simulink library "LiBatteryElements_lib"  (Simulink 7.6)
settings: Solver=ode45  StartTime=0.0  StopTime=10.0  RelTol=1e-3
undefined symbols (not defined in the file or in its folder): gcbh, nesl_callback
settings Model: Creator=rjackey  LastModifiedBy=rjackey

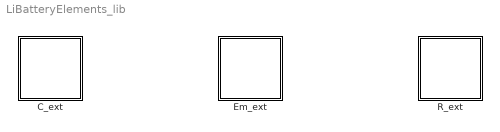
== system LiBatteryElements_lib ==
  C_ext : Subsystem  DialogController=NetworkEngine.DynNeDlgSource  LoadFcn=nesl_callback('LoadFcn',gcbh);  mask(C_ext){ComponentPath=LiBatteryElements.C_ext, ClassName=C_ext, SchemaVersion=1, v0=0, v0_unit=V, Cmin=1e-6, Cmin_unit=F, i_Log=off, v_Log=off, LocalVarNames=|i|v, LocalVarDescs=|i|v, LocalVarLogging=[0 0]}
      mask prompts: v0 "Initial voltage across capacitor"; Cmin "Minimum capacitance C>=0"
      mask help: This block implements a variable capacitance C, and assumes the capacitance does not change quickly. Copyright 2012 The MathWorks, Inc.
      mask init:
      | nesl_preinitmask (gcb);
      settings: CopyFcn=nesl_callback('CopyFcn',gcbh);  DeleteFcn=nesl_callback('DeleteFcn',gcbh);  ModelCloseFcn=nesl_callback('ModelCloseFcn',gcbh);  PreSaveFcn=nesl_callback('PreSaveFcn',gcbh);  PostSaveFcn=nesl_callback('PostSaveFcn',gcbh);  PreCopyFcn=nesl_callback('PreCopyFcn',gcbh);  PreDeleteFcn=nesl_callback('PreDeleteFcn',gcbh);
      mask Help: web(nesl_help(gcbh))
      mask Display:
      | color('blue');
      | disp('Simscape\n\n\n')
      | color('black');disp('\n\n\nC_ext');;
      | color('red');
      | port_label('LConn', 1,'+')
      | port_label('RConn', 1,'-')
      | port_label('LConn', 2,'C')
  Em_ext : Subsystem  DialogController=NetworkEngine.DynNeDlgSource  LoadFcn=nesl_callback('LoadFcn',gcbh);  mask(Em_ext){ComponentPath=LiBatteryElements.Em_ext, ClassName=Em_ext, SchemaVersion=1, Qinit=0, Qinit_unit=hr*A, i_Log=off, v_Log=off, Qe_Log=off, LocalVarNames=|i|v|Qe, LocalVarDescs=|i|v|Charge deficit, LocalVarLogging=[0 0 0]}
      mask prompts: Qinit "Initial charge deficit"
      mask help: This block implements the main branch voltage source and state of charge (SOC). Copyright 2012 The MathWorks, Inc.
      mask init:
      | nesl_preinitmask (gcb);
      settings: CopyFcn=nesl_callback('CopyFcn',gcbh);  DeleteFcn=nesl_callback('DeleteFcn',gcbh);  ModelCloseFcn=nesl_callback('ModelCloseFcn',gcbh);  PreSaveFcn=nesl_callback('PreSaveFcn',gcbh);  PostSaveFcn=nesl_callback('PostSaveFcn',gcbh);  PreCopyFcn=nesl_callback('PreCopyFcn',gcbh);  PreDeleteFcn=nesl_callback('PreDeleteFcn',gcbh);
      mask Help: web(nesl_help(gcbh))
      mask Display:
      | color('blue');
      | disp('Simscape\n\n\n')
      | color('black');disp('\n\n\nEm_ext');;
      | color('red');
      | port_label('LConn', 1,'+')
      | port_label('RConn', 1,'-')
      | port_label('RConn', 2,'V')
      | port_label('RConn', 3,'C')
      | port_label('LConn', 2,'SOC')
  R_ext : Subsystem  DialogController=NetworkEngine.DynNeDlgSource  LoadFcn=nesl_callback('LoadFcn',gcbh);  mask(R_ext){ComponentPath=LiBatteryElements.R_ext, ClassName=R_ext, SchemaVersion=1, Rmin=0, Rmin_unit=Ohm, i_Log=off, v_Log=off, LocalVarNames=|i|v, LocalVarDescs=|i|v, LocalVarLogging=[0 0]}
      mask prompts: Rmin "Minimum resistance R>=0"
      mask help: This block implements a variable polynomial resistance R. Copyright 2012 The MathWorks, Inc.
      mask init:
      | nesl_preinitmask (gcb);
      settings: CopyFcn=nesl_callback('CopyFcn',gcbh);  DeleteFcn=nesl_callback('DeleteFcn',gcbh);  ModelCloseFcn=nesl_callback('ModelCloseFcn',gcbh);  PreSaveFcn=nesl_callback('PreSaveFcn',gcbh);  PostSaveFcn=nesl_callback('PostSaveFcn',gcbh);  PreCopyFcn=nesl_callback('PreCopyFcn',gcbh);  PreDeleteFcn=nesl_callback('PreDeleteFcn',gcbh);
      mask Help: web(nesl_help(gcbh))
      mask Display:
      | color('blue');
      | disp('Simscape\n\n\n')
      | color('black');disp('\n\n\nR_ext');;
      | color('red');
      | port_label('LConn', 1,'+')
      | port_label('RConn', 1,'-')
      | port_label('LConn', 2,'R')
      | port_label('RConn', 2,'POW')

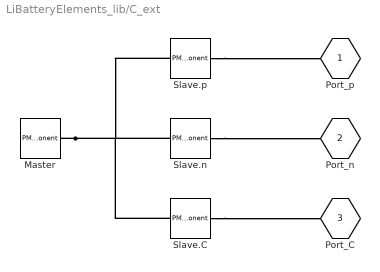
== system LiBatteryElements_lib/C_ext ==
  Master : PMComponent  Tag=LiBatteryElements.C_ext  PhysicalDomain=network_engine_domain  SubClassName=master  LeftPortType=generic  RightPortType=generic  RConnTagsString=RConn1
      mask Display: disp('Hub')
  Slave.C : PMComponent  Tag=C  PhysicalDomain=network_engine_domain  SubClassName=input  LeftPortType=generic  RightPortType=input  LConnTagsString=LConn1  RConnTagsString=RConn1
      mask Display: disp('Slave')
  Slave.n : PMComponent  Tag=n  PhysicalDomain=network_engine_domain  SubClassName=terminal  LeftPortType=generic  RightPortType=foundation.electrical.electrical  LConnTagsString=LConn1  RConnTagsString=RConn1
      mask Display: disp('Slave')
  Slave.p : PMComponent  Tag=p  PhysicalDomain=network_engine_domain  SubClassName=terminal  LeftPortType=generic  RightPortType=foundation.electrical.electrical  LConnTagsString=LConn1  RConnTagsString=RConn1
      mask Display: disp('Slave')
  Port_p : PMIOPort  Tag=p  Port=1  Side=Left
  Port_n : PMIOPort  Tag=n  Port=2  Side=Right
  Port_C : PMIOPort  Tag=C  Port=3  Side=Left
  connections:
  Slave.p/RConn1 -- Port_p/RConn1
  Slave.p/LConn1 -- Slave.n/LConn1 -- Master/RConn1 -- Slave.C/LConn1
  Slave.n/RConn1 -- Port_n/RConn1
  Slave.C/RConn1 -- Port_C/RConn1

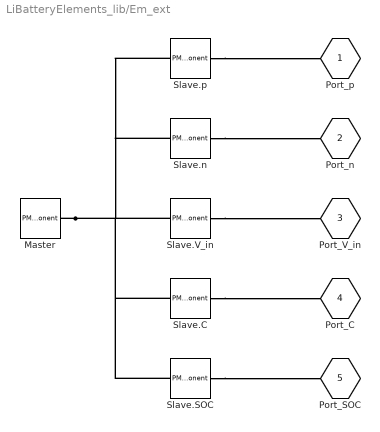
== system LiBatteryElements_lib/Em_ext ==
  Master : PMComponent  Tag=LiBatteryElements.Em_ext  PhysicalDomain=network_engine_domain  SubClassName=master  LeftPortType=generic  RightPortType=generic  RConnTagsString=RConn1
      mask Display: disp('Hub')
  Slave.C : PMComponent  Tag=C  PhysicalDomain=network_engine_domain  SubClassName=input  LeftPortType=generic  RightPortType=input  LConnTagsString=LConn1  RConnTagsString=RConn1
      mask Display: disp('Slave')
  Slave.SOC : PMComponent  Tag=SOC  PhysicalDomain=network_engine_domain  SubClassName=output  LeftPortType=generic  RightPortType=output  LConnTagsString=LConn1  RConnTagsString=RConn1
      mask Display: disp('Slave')
  Slave.V_in : PMComponent  Tag=V_in  PhysicalDomain=network_engine_domain  SubClassName=input  LeftPortType=generic  RightPortType=input  LConnTagsString=LConn1  RConnTagsString=RConn1
      mask Display: disp('Slave')
  Slave.n : PMComponent  Tag=n  PhysicalDomain=network_engine_domain  SubClassName=terminal  LeftPortType=generic  RightPortType=foundation.electrical.electrical  LConnTagsString=LConn1  RConnTagsString=RConn1
      mask Display: disp('Slave')
  Slave.p : PMComponent  Tag=p  PhysicalDomain=network_engine_domain  SubClassName=terminal  LeftPortType=generic  RightPortType=foundation.electrical.electrical  LConnTagsString=LConn1  RConnTagsString=RConn1
      mask Display: disp('Slave')
  Port_p : PMIOPort  Tag=p  Port=1  Side=Left
  Port_n : PMIOPort  Tag=n  Port=2  Side=Right
  Port_V_in : PMIOPort  Tag=V_in  Port=3  Side=Right
  Port_C : PMIOPort  Tag=C  Port=4  Side=Right
  Port_SOC : PMIOPort  Tag=SOC  Port=5  Side=Left
  connections:
  Slave.p/RConn1 -- Port_p/RConn1
  Slave.p/LConn1 -- Slave.n/LConn1 -- Slave.V_in/LConn1 -- Slave.C/LConn1 -- Master/RConn1 -- Slave.SOC/LConn1
  Slave.n/RConn1 -- Port_n/RConn1
  Slave.V_in/RConn1 -- Port_V_in/RConn1
  Slave.C/RConn1 -- Port_C/RConn1
  Slave.SOC/RConn1 -- Port_SOC/RConn1

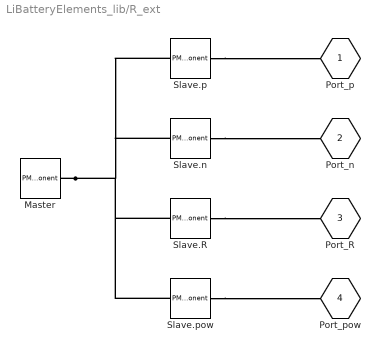
== system LiBatteryElements_lib/R_ext ==
  Master : PMComponent  Tag=LiBatteryElements.R_ext  PhysicalDomain=network_engine_domain  SubClassName=master  LeftPortType=generic  RightPortType=generic  RConnTagsString=RConn1
      mask Display: disp('Hub')
  Slave.R : PMComponent  Tag=R  PhysicalDomain=network_engine_domain  SubClassName=input  LeftPortType=generic  RightPortType=input  LConnTagsString=LConn1  RConnTagsString=RConn1
      mask Display: disp('Slave')
  Slave.n : PMComponent  Tag=n  PhysicalDomain=network_engine_domain  SubClassName=terminal  LeftPortType=generic  RightPortType=foundation.electrical.electrical  LConnTagsString=LConn1  RConnTagsString=RConn1
      mask Display: disp('Slave')
  Slave.p : PMComponent  Tag=p  PhysicalDomain=network_engine_domain  SubClassName=terminal  LeftPortType=generic  RightPortType=foundation.electrical.electrical  LConnTagsString=LConn1  RConnTagsString=RConn1
      mask Display: disp('Slave')
  Slave.pow : PMComponent  Tag=pow  PhysicalDomain=network_engine_domain  SubClassName=output  LeftPortType=generic  RightPortType=output  LConnTagsString=LConn1  RConnTagsString=RConn1
      mask Display: disp('Slave')
  Port_p : PMIOPort  Tag=p  Port=1  Side=Left
  Port_n : PMIOPort  Tag=n  Port=2  Side=Right
  Port_R : PMIOPort  Tag=R  Port=3  Side=Left
  Port_pow : PMIOPort  Tag=pow  Port=4  Side=Right
  connections:
  Slave.p/RConn1 -- Port_p/RConn1
  Slave.p/LConn1 -- Slave.n/LConn1 -- Slave.R/LConn1 -- Master/RConn1 -- Slave.pow/LConn1
  Slave.n/RConn1 -- Port_n/RConn1
  Slave.R/RConn1 -- Port_R/RConn1
  Slave.pow/RConn1 -- Port_pow/RConn1
